simulink model "task_3_sim"  (R2023a)
settings: Solver=VariableStepAuto  StartTime=0.0  StopTime=10.0  RelTol=1e-3
undefined symbols (not defined in the file): A, B, C, D, K, L, x_0, x_h_0
settings Model: Creator=user  LastModifiedBy=user

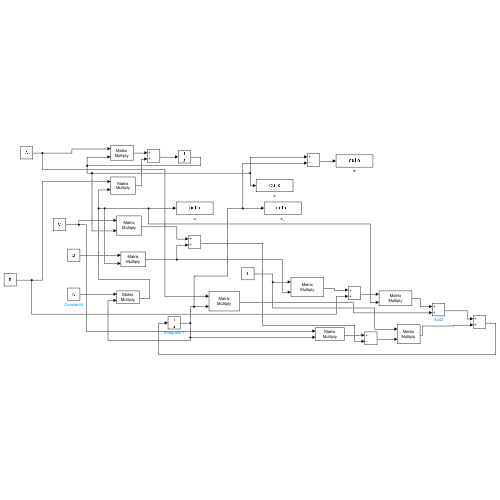
[thumbnail: Simulink's stored preview of the top-level diagram]
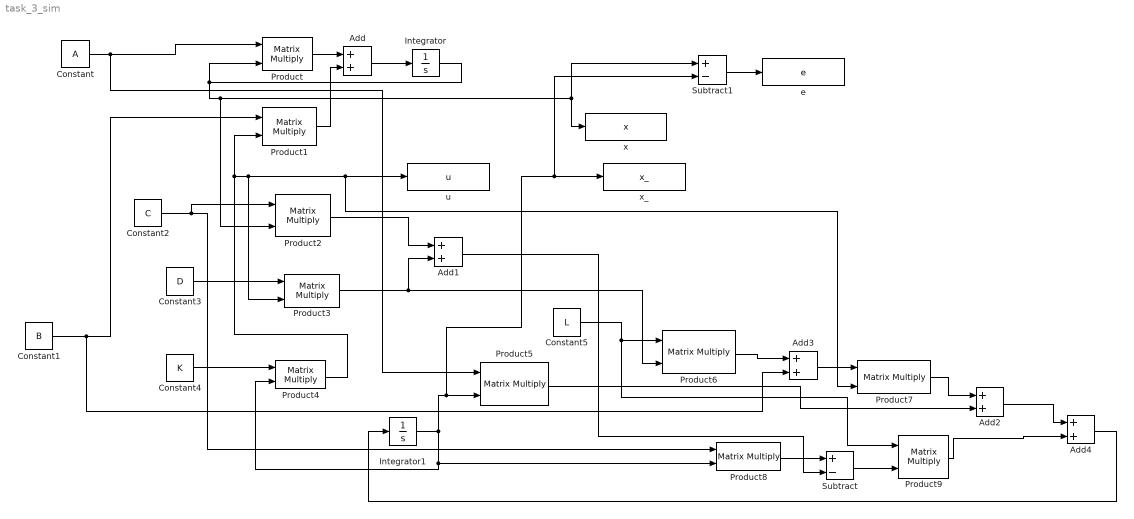
== system task_3_sim ==
  Add{,1..4} (5 alike) : Sum
  Constant : Constant  Value=A
  Constant1 : Constant  Value=B
  Constant2 : Constant  Value=C
  Constant3 : Constant  Value=D
  Constant4 : Constant  Value=K
  Constant5 : Constant  Value=L
  Integrator : Integrator  InitialCondition=x_0
  Integrator1 : Integrator  InitialCondition=x_h_0
  Product{,1..9} (10 alike) : Product  Multiplication=Matrix(*)
  Subtract : Sum  Inputs=+-
  Subtract1 : Sum  Inputs=+-
  e : ToWorkspace  VariableName=e  SaveFormat=Timeseries  SampleTime=-1
  u : ToWorkspace  VariableName=u  SaveFormat=Timeseries  SampleTime=-1
  x : ToWorkspace  VariableName=x  SaveFormat=Timeseries  SampleTime=-1
  x_ : ToWorkspace  VariableName=x_  SaveFormat=Timeseries  SampleTime=-1
  wires:
  Constant/1 -> Product5/1, Product/1
  Product/1 -> Add/1
  Constant1/1 -> Add3/2, Product1/1
  Product4/1 -> Product1/2, Product3/2, Product7/2, u/1
  Product1/1 -> Add/2
  Add/1 -> Integrator/1
  Constant2/1 -> Product8/1, Product2/1
  Constant3/1 -> Product3/1
  Product2/1 -> Add1/1
  Product3/1 -> Product6/2, Add1/2
  Constant4/1 -> Product4/1
  Integrator1/1 -> Product8/2, Product4/2, Subtract1/2, x_/1, Product5/2
  Constant5/1 -> Product9/1, Product6/1
  Product6/1 -> Add3/1
  Add3/1 -> Product7/1
  Product7/1 -> Add2/1
  Product5/1 -> Add2/2
  Add2/1 -> Add4/1
  Product8/1 -> Subtract/1
  Add1/1 -> Subtract/2
  Subtract/1 -> Product9/2
  Product9/1 -> Add4/2
  Add4/1 -> Integrator1/1
  Integrator/1 -> Product2/2, x/1, Subtract1/1, Product/2
  Subtract1/1 -> e/1
